simulink model "rezervoar_nelinearni"  (R2016a)
settings: Solver=VariableStepAuto  StartTime=0.0  StopTime=1000.0  RelTol=1e-3
values from neighbouring files (symbols this model uses):
  A0 = 0.01    [postavljanje_konstanti.m]
  A1 = 2    [postavljanje_konstanti.m]
  g = 9.81    [postavljanje_konstanti.m]
  qu_max = 0.099    [postavljanje_konstanti.m]
settings Model: Creator=Vukan  LastModifiedBy=Vukan

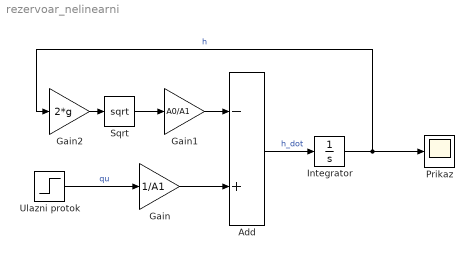
== system rezervoar_nelinearni ==
  Add : Sum  Inputs=-+
  Gain : Gain  Gain=1/A1
  Gain1 : Gain  Gain=A0/A1
  Gain2 : Gain  Gain=2*g
  Integrator : Integrator
  Prikaz : Scope
  Sqrt : Sqrt  SaturateOnIntegerOverflow=on
  Ulazni protok : Step  Time=100  After=qu_max  SampleTime=0
  wires:
  Ulazni protok/1 -> Gain/1  "qu"
  Gain/1 -> Add/2
  Add/1 -> Integrator/1  "h_dot"
  Integrator/1 -> Gain2/1, Prikaz/1  "h"
  Sqrt/1 -> Gain1/1
  Gain2/1 -> Sqrt/1
  Gain1/1 -> Add/1
